simulink model "ripple"  (R2015a)
settings: Solver=ode3  StartTime=0.0  StopTime=10.0  RelTol=1e-3
settings Model: Creator=thaodang  LastModifiedBy=thaodang

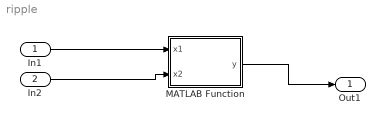
== system ripple ==
  In1 : Inport  OutDataTypeStr=double
  In2 : Inport  Port=2  OutDataTypeStr=double
  MATLAB Function : MATLAB Function  TreatAsAtomicUnit=on
  Out1 : Outport
  wires:
  In1/1 -> MATLAB Function/1(x1)
  In2/1 -> MATLAB Function/2(x2)
  MATLAB Function/1(y) -> Out1/1

== matlab function ripple/MATLAB Function ==
  data: x1 input; y output; x2 input
function y = fcn(x1, x2)
%#codegen

%pi=3.14;

res1 = - exp( - 2*log(2)*((x1 - 0.1)/0.8)^2 ) * ((sin(5*pi*x1))^6 + 0.1*( cos(500*pi*x1))^2 );
y = res1 - exp( - 2*log(2)*((x2 - 0.1)/0.8)^2 ) * (( sin(5*pi*x2))^6 + 0.1*(cos(500*pi*x2))^2 );
